simulink subsystem "sim_bridge"  (R2025b)
settings: Solver=VariableStepAuto  StartTime=0.0  StopTime=10.0  RelTol=1e-3
libraries: simulink x3, svdutilitieslib x2, c280xlib x2
settings Model: Creator=erik  LastModifiedBy=erik

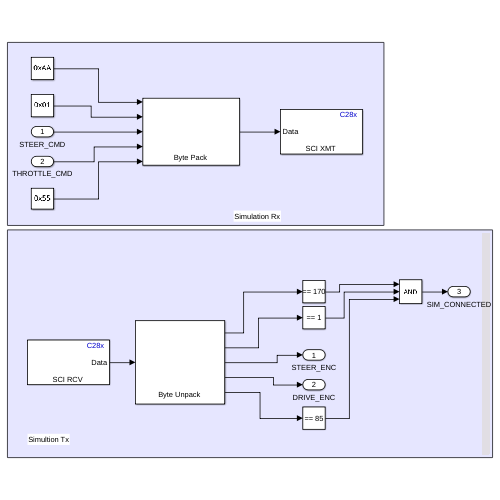
[thumbnail: Simulink's stored preview of the top-level diagram]
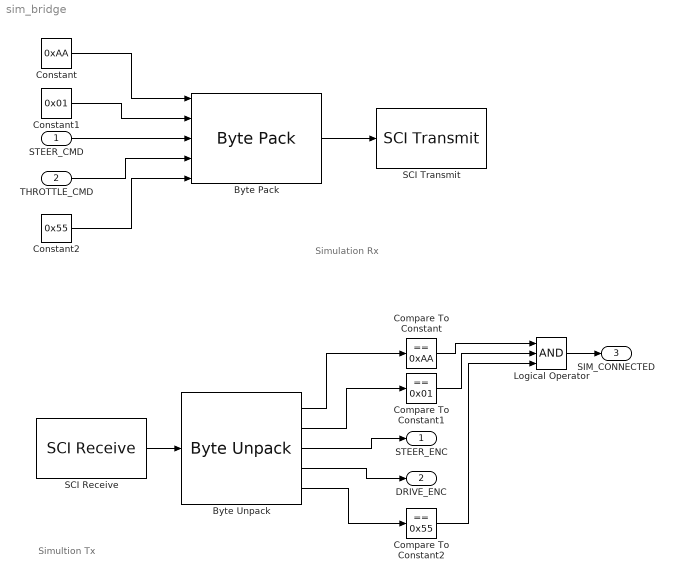
== system sim_bridge ==
  note: Simulation Rx
  note: Simultion Tx
  STEER_CMD : Inport
  THROTTLE_CMD : Inport  Port=2
  Byte Pack : svdutilitieslib/Byte Pack  maskPackedDataType=uint8  datatypes={'uint8','uint8','int16','int16','uint8'}  byteAlign=1  blockPlatform=tic2000
      settings: LibrarySourceBlock=c2000lib/Target Communication/Byte Pack
  Byte Unpack : svdutilitieslib/Byte Unpack  dimensions={[1],[1],[1],[1],[1]}  datatypes={'uint8','uint8','int32','int32','uint8'}  byteAlign=1  blockPlatform=tic2000
      settings: LibrarySourceBlock=c2000lib/Target Communication/Byte Unpack
  Compare To Constant : simulink/Logic and Bit Operations/Compare To Constant  relop===  const=0xAA  OutDataTypeStr=boolean
  Compare To Constant1 : simulink/Logic and Bit Operations/Compare To Constant  relop===  const=0x01  OutDataTypeStr=boolean
  Compare To Constant2 : simulink/Logic and Bit Operations/Compare To Constant  relop===  const=0x55  OutDataTypeStr=boolean
  Constant : Constant  Value=0xAA
  Constant1 : Constant  Value=0x01
  Constant2 : Constant  Value=0x55
  Logical Operator : Logic  Inputs=3  AllPortsSameDT=off  OutDataTypeStr=boolean
  SCI Receive : c280xlib/SCI Receive  Priority=2  sciModule=B  dataHead=''  headerCheckMaxCount=16  dataTail=''  dataType=uint8  dataLenOptions=Length via dialog  dataDim=12  maxDataLength=1  initValue=0  errOption=Output custom value  errValue=0  sampleTime=0.1  blockingMode=on  timeOut=inf  outputStatus=off
      settings: LibrarySourceBlock=c2837xDlib/SCI Receive
  SCI Transmit : c280xlib/SCI Transmit  sciModule=B  dataHead=''  dataTail=''  frameSize=8  blockingMode=on  outputStatus=off
      settings: LibrarySourceBlock=c2837xDlib/SCI Transmit
  STEER_ENC : Outport
  DRIVE_ENC : Outport  Port=2
  SIM_CONNECTED : Outport  Port=3
  wires:
  Constant/1 -> Byte Pack/1
  Constant1/1 -> Byte Pack/2
  STEER_CMD/1 -> Byte Pack/3
  THROTTLE_CMD/1 -> Byte Pack/4
  Constant2/1 -> Byte Pack/5
  Byte Pack/1 -> SCI Transmit/1
  SCI Receive/1 -> Byte Unpack/1
  Byte Unpack/3 -> STEER_ENC/1
  Byte Unpack/4 -> DRIVE_ENC/1
  Byte Unpack/1 -> Compare To Constant/1
  Byte Unpack/2 -> Compare To Constant1/1
  Byte Unpack/5 -> Compare To Constant2/1
  Compare To Constant/1 -> Logical Operator/1
  Compare To Constant1/1 -> Logical Operator/2
  Compare To Constant2/1 -> Logical Operator/3
  Logical Operator/1 -> SIM_CONNECTED/1
